simulink model "twoaxis_camera_gantry_start_work_project_Yejesh_final"  (R2025b)
settings: Solver=ode15s  StartTime=0.0  StopTime=60  MaxStep=1e-3  RelTol=1e-3  EnableMultiTasking=on
model workspace: external: MATLAB File gantryParams.m (data not in the file)
undefined symbols (not defined in the file): endSupport, endSupportZ, fractalcoef, leadScrew, leadScrewZ, rail, railZ, runner, runnerZ, X, Y, Z
libraries: sm_lib x81, nesl_utility x14, sm_linear_actuator_lib x14, fl_lib x6, slpidlib x2, mspsensorlib x1
(part 1 of 4)
Description:
  | Using the Lead Screw Joint Block - Linear Actuator
  | 
  | This example illustrates the use of the Lead Screw Joint block to model a linear actuator. The Lead
  | Screw Joint block converts rotational motion at the Revolute Joint block to translational motion at
  | the four Cylindrical Joint blocks. The translational motion is specified as a motion input to a
  | cylindrical joint and the necessary actuator torque is automatically computed at the revolute joint.
settings Model: PacingRate=4  Creator=The MathWorks, Inc.  LastModifiedBy=yejes
settings SolverCC: AlgebraicLoopSolver=TrustRegion
settings DataIOCC: LimitDataPoints=on  SaveFormat=Array  ReturnWorkspaceOutputs=off
settings OptimizationCC: LifeSpan=inf
settings DebuggingCC: SolverPrmCheckMsg=warning  UnconnectedInputMsg=warning  UnconnectedOutputMsg=warning  UnconnectedLineMsg=warning  AllowSymbolicDim=off  SFUnexpectedBacktrackingDiag=warning  SFNoUnconditionalDefaultTransitionDiag=warning  SFExecutionAtInitializationDiag=none  ArithmeticOperatorsInVariantConditions=warning
settings HardwareCC: ProdBitPerPointer=32.0  ProdBitPerSizeT=32.0  ProdBitPerPtrDiffT=32.0  ProdLargestAtomicFloat=None  ProdIntDivRoundTo=Undefined  ProdEndianess=Unspecified  ProdWordSize=32.0  ProdHWDeviceType=32-bit Generic
settings ModelReferenceCC: EnableRefExpFcnMdlSchedulingChecks=on  PropagateSignalLabelsOutOfModel=off
settings SFSimCC: SimUseLocalCustomCode=off  CustomCodeUndefinedFunction=UseInterfaceOnly
settings RTWCC: RTWUseLocalCustomCode=off  GPUComputeCapability=3.5  DLArmComputeVersion=19.05
settings CodeAppCC: StateflowObjectComments=on
settings GRTTargetCC: TargetLangStandard=C89/C90 (ANSI)
settings ConfigComp: CovMetricSettings=dw  CovSaveCumulativeToWorkspaceVar=on  CovSaveSingleToWorkspaceVar=on  CovExternalEMLEnable=off  CovSFcnEnable=off
settings SimscapeCC: SimscapeNormalizeSystem=off
settings ConfigurationSet: Description=SimMechanics 2G
settings DiagnosticsConfigSet: SimMechanicsUnconnectedFramePorts=none
settings ExplorerConfigSet: InternalSimMechanicsExplorerSettings="<ExplorerConfiguration><canonicalview>default</canonicalview><AnimationSetting><BasePlaybackSpeed>1.0</BasePlaybackSpeed><PlaybackSpeedFactor>1.0</PlaybackSpeedFactor></AnimationSetting><TilePanel><TileInfo><Tiles Columns=\"1\" Count=\"1\" Rows=\"1\"><Column Weight=\"1\"/><Row Weight=\"1\"/><Tile Height=\"1\" Width=\"1\" X=\"0\" Y=\"0\"/></Tiles></TileInfo><SceneInfo><SceneViewer><BGColor><R>1</R><G>1</G><B>1</B></BGColor><Camera><DoPerspective>off</DoPerspective><Position><X>0.577350260811389404</X><Y>-0.277350261388458308</Y><Z>0.937350262073923357</Z></Position><Center><X>-8.37823641020030152e-09</X><Y>0.300000007801167534</Y><Z>0.35999999288429757</Z></Center><Up><X>-0.408248290463863073</X><Y>0.408248290463863073</Y><Z>0.816496580927726145</Z></Up><ViewLimDist>1</ViewLimDist><YLim>0.483570086956024159</YLim><XLim>0.367001870038164535</XLim></Camera></SceneViewer></SceneInfo></TilePanel><MechEditorPanel><Cameras/><GfxPanelCameraMap/><VideoCreator><PlaybackSpeedRatio>1.0</PlaybackSpeedRatio><FrameRate>30</FrameRate><VideoFormat>Motion JPEG AVI</VideoFormat><FrameSize>auto</FrameSize></VideoCreator></MechEditorPanel></ExplorerConfiguration>"

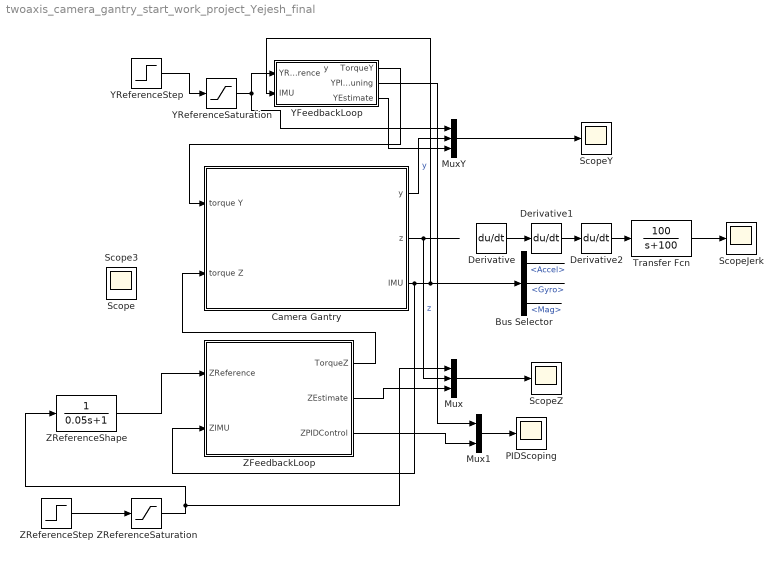
== system twoaxis_camera_gantry_start_work_project_Yejesh_final ==
  "\tCamera Gantry" : Subsystem
      mask Display: image('$imagefile'); % Use "Edit Image" on toolstrip to change.
  Bus Selector : BusSelector  OutputSignals=Accel,Gyro,Mag
  Derivative : Derivative
  Derivative1 : Derivative
  Derivative2 : Derivative
  Mux : Mux  Inputs=3
  Mux1 : Mux  Inputs=2
  MuxY : Mux  Inputs=3
  PIDScoping : Scope
      settings: ActiveDisplayYMinimum=-23.035365801646694  ActiveDisplayYMaximum=17.371677932919315  DataLoggingVariableName=ScopeData8
  ScopeJerk : Scope
  ScopeY : Scope
      settings: ActiveDisplayYMinimum=-0.074128762499999987  ActiveDisplayYMaximum=0.6671588625  DataLoggingVariableName=ScopeData2
  ScopeZ : Scope
      settings: ActiveDisplayYMinimum=-0.14165423833378787  ActiveDisplayYMaximum=0.64811641951018473  DataLoggingVariableName=ScopeData3
  Transfer Fcn : TransferFcn  Numerator=[100]  Denominator=[1 100]
  YFeedbackLoop : Subsystem
      settings: PortSchema="{\"entries\":[{\"content\":{\"sides\":[{\"content\":{\"connectorIds\":[\"In1\",\"In2\"]},\"type\":\"ConnectorPlacement.EquallySpacedRectSide\",\"uuid\":\"2f6c7822-fa00-4de6-9e32-64451994c035\"},{\"content\":{\"connectorIds\":[\"Out1\",\"Out2\",\"Out3\"],\"side\":\"RIGHT\"},\"type\":\"ConnectorPlacement.EquallySpacedRectSide\",\"uuid\":\"522d5529-44ef-4061-9e28-ddd46f5bc78d\"},{\"content\":{\"connectorIds\":[\"In3\"],\"side\":\"TOP\"},\"type\":\"ConnectorPlacement.EquallySpacedRectSide\",\"uuid\":\"f2a467b7-c03a-4305-9c34-f8fdeacd5866\"}]},\"type\":\"ConnectorPlacement.EquallySpacedConnector\",\"uuid\":\"6b65950b-cfc7-46ba-97f3-5f54aada1479\"}],\"packageUris\":[\"http://schema.mathworks.com/mf0/Connector/R2020b\"],\"version\":\"1.0\"}"
  YReferenceSaturation : Saturate  UpperLimit=0.75  LowerLimit=0
  YReferenceStep : Step  Time=0.5  Before=0.3  After=0.35  SampleTime=0
  ZFeedbackLoop : Subsystem
  ZReferenceSaturation : Saturate  UpperLimit=0.4  LowerLimit=0
  ZReferenceShape : TransferFcn  Denominator=[0.05 1]
  ZReferenceStep : Step  Time=0.5  Before=0.20  After=0.25  SampleTime=0
  Scope : Scope
      settings: ActiveDisplayYMinimum=-5.6117722223923652  ActiveDisplayYMaximum=5.5774668558867786  DataLoggingVariableName=ScopeData4
  Scope3 : Scope
      settings: ActiveDisplayYMinimum=0.1911  ActiveDisplayYMaximum=0.2439
  wires:
  "\tCamera Gantry"/3(IMU) -> ZFeedbackLoop/2(ZIMU), YFeedbackLoop/2(IMU), Bus Selector/1
  Bus Selector/1 -> ?  "<Accel>"
  Bus Selector/2 -> ?  "<Gyro>"
  Bus Selector/3 -> ?  "<Mag>"
  "\tCamera Gantry"/2(z) -> Mux/2  "z"
  YReferenceStep/1 -> YReferenceSaturation/1
  YReferenceSaturation/1 -> YFeedbackLoop/1(YReference), MuxY/1
  ZReferenceStep/1 -> ZReferenceSaturation/1
  ZReferenceSaturation/1 -> Mux/1, ZReferenceShape/1
  YFeedbackLoop/1(TorqueY) -> "\tCamera Gantry"/1(torque Y)
  ZReferenceShape/1 -> ZFeedbackLoop/1(ZReference)
  ZFeedbackLoop/1(TorqueZ) -> "\tCamera Gantry"/2(torque Z)
  Derivative/1 -> Derivative1/1
  Derivative1/1 -> Derivative2/1
  Derivative2/1 -> Transfer Fcn/1
  Transfer Fcn/1 -> ScopeJerk/1
  "\tCamera Gantry"/1(y) -> MuxY/2  "y"
  YFeedbackLoop/3(YEstimate) -> MuxY/3
  MuxY/1 -> ScopeY/1
  Mux/1 -> ScopeZ/1
  ZFeedbackLoop/2(ZEstimate) -> Mux/3
  Mux1/1 -> PIDScoping/1
  ZFeedbackLoop/3(ZPIDControl) -> Mux1/2
  YFeedbackLoop/2(YPIDTuning) -> Mux1/1

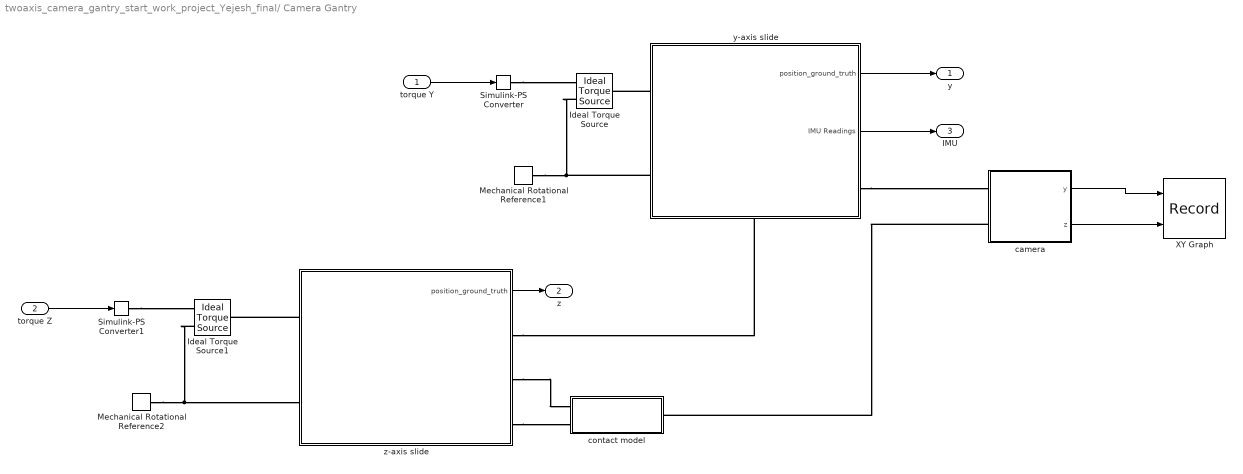
== system twoaxis_camera_gantry_start_work_project_Yejesh_final/	Camera Gantry ==
  torque Y : Inport
  torque Z : Inport  Port=2
  Ideal Torque Source : fl_lib/Mechanical/Mechanical Sources/Ideal Torque Source
  Ideal Torque Source1 : fl_lib/Mechanical/Mechanical Sources/Ideal Torque Source
  Mechanical Rotational Reference1 : fl_lib/Mechanical/Rotational Elements/Mechanical Rotational Reference
  Mechanical Rotational Reference2 : fl_lib/Mechanical/Rotational Elements/Mechanical Rotational Reference
  Simulink-PS Converter : nesl_utility/Simulink-PS Converter  PhysicalDomain=network_engine_domain  SubClassName=ps_input  LeftPortType=input  RightPortType=output  PseudoPeriodic=off  Frequencies=[]  NoiseDistribution=none  NoiseParameters=[]  Unit=1  AffineConversion=off  FilteringAndDerivatives=provide  SimscapeFilterOrder=1  InputFilterTimeConstant=0.001  UdotUserProvided=0
  Simulink-PS Converter1 : nesl_utility/Simulink-PS Converter  PhysicalDomain=network_engine_domain  SubClassName=ps_input  LeftPortType=input  RightPortType=output  PseudoPeriodic=off  Frequencies=[]  NoiseDistribution=none  NoiseParameters=[]  Unit=1  AffineConversion=off  FilteringAndDerivatives=provide  SimscapeFilterOrder=1  InputFilterTimeConstant=0.001  UdotUserProvided=0
  XY Graph : Record  NumPorts=2.0  FileSettingsInternal="{\"entries\":[{\"content\":{\"excelSettings\":{\"content\":{},\"type\":\"Streamout.ExcelSettings\"},\"parquetSettings\":{\"content\":{},\"type\":\"Streamout.ParquetSettings\"}},\"type\":\"Streamout.FileSettingStorage\",\"uuid\":\"\"}],\"packageUris\":[\"http:\\/\\/schema.mathworks.com\\/mf0\\/streamout_blocks\\/R2020a\"],\"version\":\"1.0\"}"  FrameSettings=[0, 0]  Layout=[1 1]  SignalsInternal="{\"entries\":[{\"content\":{\"signals\":[{\"content\":{\"blockPath\":[],\"dimensions\":[1],\"domain\":\"\",\"lineColor\":\"#a2142f\",\"plots\":[ 1 ],\"port\":1,\"sid\":[\"\"],\"signalID\":1,\"signalName\":\"camera:1\"},\"type\":\"RecordBlkView.Signal\",\"uuid\":\"\"},{\"content\":{\"blockPath\":[],\"dimensions\":[1],\"domain\":\"\",\"lineColor\":\"#139fff\",\"plots\":[ 1 ],\"port\":2,\"sid\":[\"\"],\"signalID\":2,\"signalName\":\"camera:2\"},\"type\":\"RecordBlkView.Signal\",\"uuid\":\"\"}]},\"type\":\"RecordBlkView.InputSignals\",\"uuid\":\"\"}],\"packageUris\":[\"http:\\/\\/schema.mathworks.com\\/mf0\\/streamout_blocks\\/R2020a\"],\"version\":\"1.0\"}"  VisualizationBindings="{\"xyplotplugin\":{\"info\":[{\"series\":[{\"bindingParametersList\":[{\"parameter\":\"X-Axis\",\"signalID\":1,\"signalName\":\"camera:1\"},{\"parameter\":\"Y-Axis\",\"signalID\":2,\"signalName\":\"camera:2\"}],\"seriesID\":0}],\"subplotID\":1}]}}"  CompatibilityTag=XY
  camera : Subsystem
      mask Display: image('$imagefile'); % Use "Edit Image" on toolstrip to change.
  contact model : Subsystem
  y-axis slide : Subsystem
      settings: PortSchema="{\"entries\":[{\"content\":{\"sides\":[{\"content\":{\"connectorIds\":[\"LConn1\",\"LConn2\"]},\"type\":\"ConnectorPlacement.EquallySpacedRectSide\",\"uuid\":\"3f377b63-bc87-4e06-8b63-1d64c166b4f3\"},{\"content\":{\"connectorIds\":[\"Out1\",\"Out2\",\"RConn1\"],\"side\":\"RIGHT\"},\"type\":\"ConnectorPlacement.EquallySpacedRectSide\",\"uuid\":\"3affb14a-8bdc-4f8f-893e-0f417901967e\"},{\"content\":{\"connectorIds\":[],\"side\":\"TOP\"},\"type\":\"ConnectorPlacement.EquallySpacedRectSide\",\"uuid\":\"c82e62d7-ab85-41ce-b1ad-21607245c47e\"},{\"content\":{\"connectorIds\":[\"RConn2\"],\"side\":\"BOTTOM\"},\"type\":\"ConnectorPlacement.EquallySpacedRectSide\",\"uuid\":\"9d54362b-4991-4bea-87e6-d83ba5b68b2b\"}]},\"type\":\"ConnectorPlacement.EquallySpacedConnector\",\"uuid\":\"4017ed31-76af-4f0f-8b41-874461299965\"}],\"packageUris\":[\"http://schema.mathworks.com/mf0/Connector/R2020b\"],\"version\":\"1.0\"}"
      mask Display: image('$imagefile'); % Use "Edit Image" on toolstrip to change.
  z-axis slide : Subsystem
      mask Display: image('$imagefile'); % Use "Edit Image" on toolstrip to change.
  y : Outport
  z : Outport  Port=2
  IMU : Outport  Port=3
  wires:
  camera/1(y) -> XY Graph/1
  y-axis slide/1(position_ground_truth) -> y/1
  y-axis slide/2(IMU Readings) -> IMU/1
  z-axis slide/1(position_ground_truth) -> z/1
  camera/2(z) -> XY Graph/2
  torque Y/1 -> Simulink-PS Converter/1
  torque Z/1 -> Simulink-PS Converter1/1
  connections:
  y-axis slide/LConn1 -- Ideal Torque Source/LConn1
  y-axis slide/RConn1 -- camera/LConn1
  z-axis slide/LConn1 -- Ideal Torque Source1/LConn1
  Ideal Torque Source1/RConn2 -- Mechanical Rotational Reference2/LConn1 -- z-axis slide/LConn2
  z-axis slide/RConn1 -- y-axis slide/RConn2
  z-axis slide/RConn2 -- contact model/LConn1
  z-axis slide/RConn3 -- contact model/LConn2
  camera/LConn2 -- contact model/RConn1
  Mechanical Rotational Reference1/LConn1 -- Ideal Torque Source/RConn2 -- y-axis slide/LConn2
  Simulink-PS Converter/RConn1 -- Ideal Torque Source/RConn1
  Simulink-PS Converter1/RConn1 -- Ideal Torque Source1/RConn1

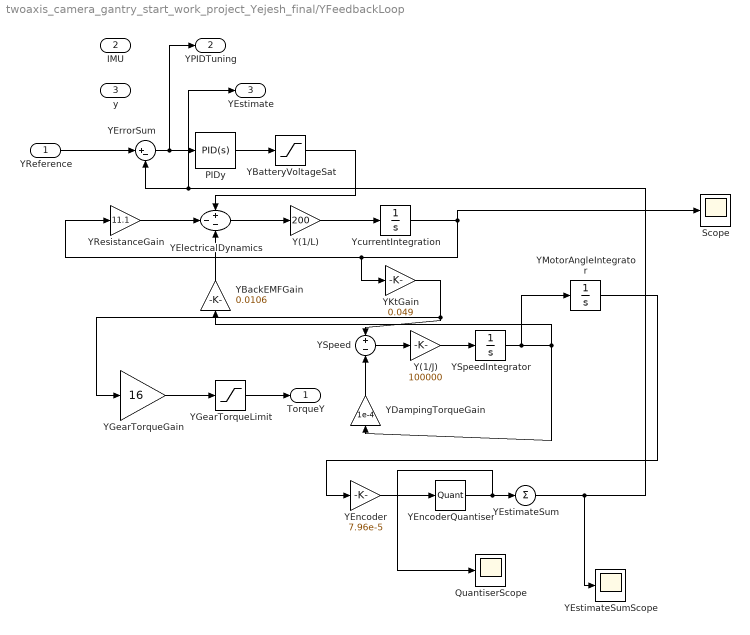
== system twoaxis_camera_gantry_start_work_project_Yejesh_final/YFeedbackLoop ==
  YReference : Inport
  IMU : Inport  Port=2
  y : Inport  Port=3
  PIDy : slpidlib/PID Controller  Controller=PID  Form=Parallel  TimeDomain=Continuous-time  UseExternalTs=off  SampleTime=-1  IntegratorMethod=Forward Euler  FilterMethod=Forward Euler  ControllerParametersSource=internal  P=30  I=10  UseKiTs=off  D=2  UseExternalDerivativeSource=off  N=100  UseFilter=on  TunerSelectOption=Transfer Function Based (PID Tuner App)  InitialConditionSource=internal  InitialConditionForIntegrator=0  InitialConditionForFilter=0  DifferentiatorICPrevScaledInput=0  ExternalReset=none  TrackingMode=off  Kt=1  LimitOutput=off  SatLimitsSource=internal  UpperSaturationLimit=inf  LowerSaturationLimit=-inf  LinearizeAsGain=on  AntiWindupMode=none  Kb=1  LimitIntegrator=off  UpperIntegratorSaturationLimit=inf  LowerIntegratorSaturationLimit=-inf  POutMin=[]  POutMax=[]  IOutMin=[]  IOutMax=[]  DOutMin=[]  DOutMax=[]  NOutMin=[]  NOutMax=[]  SumOutMin=[]  SumOutMax=[]  SaturationOutMin=[]  SaturationOutMax=[]  PParamMin=[]  PParamMax=[]  IParamMin=[]  IParamMax=[]  DParamMin=[]  DParamMax=[]  NParamMin=[]  NParamMax=[]  KbParamMin=[]  KbParamMax=[]  KtParamMin=[]  KtParamMax=[]  KbOutMin=[]  KbOutMax=[]  KtOutMin=[]  KtOutMax=[]  IntegratorOutMin=[]  IntegratorOutMax=[]  FilterOutMin=[]  FilterOutMax=[]  SumI1OutMin=[]  SumI1OutMax=[]  SumI2OutMin=[]  SumI2OutMax=[]  SumI3OutMin=[]  SumI3OutMax=[]  SumI4OutMin=[]  SumI4OutMax=[]  SumDOutMin=[]  SumDOutMax=[]  DifferentiatorOutMin=[]  DifferentiatorOutMax=[]  FilterDiffOutCoefMin=[]  FilterDiffOutCoefMax=[]  ReciprocalOutMin=[]  ReciprocalOutMax=[]  SumDenOutMin=[]  SumDenOutMax=[]  SumNumOutMin=[]  SumNumOutMax=[]  DivideOutMin=[]  DivideOutMax=[]  UdiffTsProdOutMin=[]  UdiffTsProdOutMax=[]  NTsProdOutMin=[]  NTsProdOutMax=[]  UintegralTsProdOutMin=[]  UintegralTsProdOutMax=[]  UngainTsProdOutMin=[]  UngainTsProdOutMax=[]  ClampingZeroOutDataTypeStr=Inherit: Inherit via back propagation  ClampingZeroOutMin=[]  ClampingZeroOutMax=[]  FilterDenConstantOutDataTypeStr=Inherit: Inherit via back propagation  FilterDenConstantOutMin=[]  FilterDenConstantOutMax=[]  PCopyOutDataTypeStr=Inherit: Inherit via back propagation  PCopyOutMin=[]  PCopyOutMax=[]  NCopyOutDataTypeStr=Inherit: Inherit via back propagation  NCopyOutMin=[]  NCopyOutMax=[]  IntegratorContinuousStateAttributes=''  IntegratorStateMustResolveToSignalObject=off  IntegratorRTWStateStorageClass=Auto  FilterContinuousStateAttributes=''  FilterStateMustResolveToSignalObject=off  FilterRTWStateStorageClass=Auto  ParallelPVariant=InternalParameters  IdealPVariant=Disabled  IVariant=InternalParameters  DVariant=InternalParameters  IntegratorVariant=Continuous  SatVariant=Disabled  AWVariant=Passthrough  PCopyVariant=Disabled  TRVariant=Disabled  FdbkBlocksVariant=Forward  IdealPFdbkVariant=Disabled  SatFdbkVariant=Disabled  DerivativeFilterVariant=ContFilter  NVariant=InternalParameters  NCopyVariant=Disabled  FilterICVariant=InternalICsFilter  IntegratorICVariant=InternalICs  ExternalResetVariant=Disabled  TRSumVariant=Passthrough  SumFdbkVariant=Disabled  SumVariant=Sum_PID  TsampFilterVariant=InternalTs  TsampNgainVariant=Passthrough  TsampIntegralVariant=Disabled_SignalSpec  ExternalSaturationOutDataTypeStr=Inherit: Same as second input  DerivativeSourceVariant=ErrorSignal  PreIntVariant=InternalPreInt
  QuantiserScope : Scope
      settings: DataLoggingVariableName=ScopeData5
  Scope : Scope
      settings: ActiveDisplayYMinimum=-0.89118502896327889  ActiveDisplayYMaximum=1.198287194267555  DataLoggingVariableName=ScopeData7
  Y(1/J) : Gain  Gain=100000
  Y(1/L) : Gain  Gain=200
  YBackEMFGain : Gain  Gain=0.0106
  YBatteryVoltageSat : Saturate  UpperLimit=11.1  LowerLimit=-11.1
  YDampingTorqueGain : Gain  Gain=1e-4
  YElectricalDynamics : Sum  Inputs=+--
  YEncoder : Gain  Gain=7.96e-5
  YEncoderQuantiser : Quantizer  QuantizationInterval=2.083e-5
  YErrorSum : Sum  Inputs=|+-
  YEstimateSum : Sum  Inputs=+
  YEstimateSumScope : Scope
      settings: ActiveDisplayYMinimum=-8.828451733084659  ActiveDisplayYMaximum=8.4483002375448635  DataLoggingVariableName=ScopeData6
  YGearTorqueGain : Gain  Gain=16
  YGearTorqueLimit : Saturate  UpperLimit=0.784  LowerLimit=-0.784
  YKtGain : Gain  Gain=0.049
  YMotorAngleIntegrator : Integrator
  YResistanceGain : Gain  Gain=11.1
  YSpeed : Sum  Inputs=+-
  YSpeedIntegrator : Integrator
  YcurrentIntegration : Integrator
  TorqueY : Outport
  YPIDTuning : Outport  Port=2
  YEstimate : Outport  Port=3
  wires:
  YElectricalDynamics/1 -> Y(1/L)/1
  YcurrentIntegration/1 -> YResistanceGain/1, YKtGain/1, Scope/1
  YBackEMFGain/1 -> YElectricalDynamics/3
  YResistanceGain/1 -> YElectricalDynamics/2
  YSpeedIntegrator/1 -> YDampingTorqueGain/1, YBackEMFGain/1, YMotorAngleIntegrator/1
  YKtGain/1 -> YGearTorqueGain/1, YSpeed/1
  YErrorSum/1 -> YPIDTuning/1, PIDy/1
  YBatteryVoltageSat/1 -> YElectricalDynamics/1
  PIDy/1 -> YBatteryVoltageSat/1
  Y(1/J)/1 -> YSpeedIntegrator/1
  Y(1/L)/1 -> YcurrentIntegration/1
  YDampingTorqueGain/1 -> YSpeed/2
  YSpeed/1 -> Y(1/J)/1
  YReference/1 -> YErrorSum/1
  YGearTorqueGain/1 -> YGearTorqueLimit/1
  YGearTorqueLimit/1 -> TorqueY/1
  YMotorAngleIntegrator/1 -> YEncoder/1
  YEncoder/1 -> YEncoderQuantiser/1
  YEncoderQuantiser/1 -> QuantiserScope/1, YEstimateSum/1
  YEstimateSum/1 -> YEstimateSumScope/1, YEstimate/1, YErrorSum/2

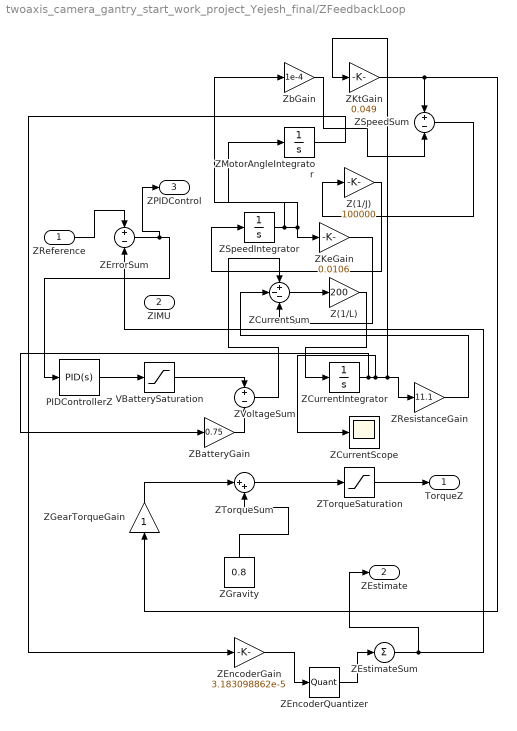
== system twoaxis_camera_gantry_start_work_project_Yejesh_final/ZFeedbackLoop ==
  ZReference : Inport
  ZIMU : Inport  Port=2
  PIDControllerZ : slpidlib/PID Controller  Controller=PID  Form=Parallel  TimeDomain=Continuous-time  UseExternalTs=off  SampleTime=-1  IntegratorMethod=Forward Euler  FilterMethod=Forward Euler  ControllerParametersSource=internal  P=50  I=30  UseKiTs=off  D=2  UseExternalDerivativeSource=off  N=100  UseFilter=on  TunerSelectOption=Transfer Function Based (PID Tuner App)  InitialConditionSource=internal  InitialConditionForIntegrator=0  InitialConditionForFilter=0  DifferentiatorICPrevScaledInput=0  ExternalReset=none  TrackingMode=off  Kt=1  LimitOutput=off  SatLimitsSource=internal  UpperSaturationLimit=inf  LowerSaturationLimit=-inf  LinearizeAsGain=on  AntiWindupMode=none  Kb=1  LimitIntegrator=off  UpperIntegratorSaturationLimit=inf  LowerIntegratorSaturationLimit=-inf  POutMin=[]  POutMax=[]  IOutMin=[]  IOutMax=[]  DOutMin=[]  DOutMax=[]  NOutMin=[]  NOutMax=[]  SumOutMin=[]  SumOutMax=[]  SaturationOutMin=[]  SaturationOutMax=[]  PParamMin=[]  PParamMax=[]  IParamMin=[]  IParamMax=[]  DParamMin=[]  DParamMax=[]  NParamMin=[]  NParamMax=[]  KbParamMin=[]  KbParamMax=[]  KtParamMin=[]  KtParamMax=[]  KbOutMin=[]  KbOutMax=[]  KtOutMin=[]  KtOutMax=[]  IntegratorOutMin=[]  IntegratorOutMax=[]  FilterOutMin=[]  FilterOutMax=[]  SumI1OutMin=[]  SumI1OutMax=[]  SumI2OutMin=[]  SumI2OutMax=[]  SumI3OutMin=[]  SumI3OutMax=[]  SumI4OutMin=[]  SumI4OutMax=[]  SumDOutMin=[]  SumDOutMax=[]  DifferentiatorOutMin=[]  DifferentiatorOutMax=[]  FilterDiffOutCoefMin=[]  FilterDiffOutCoefMax=[]  ReciprocalOutMin=[]  ReciprocalOutMax=[]  SumDenOutMin=[]  SumDenOutMax=[]  SumNumOutMin=[]  SumNumOutMax=[]  DivideOutMin=[]  DivideOutMax=[]  UdiffTsProdOutMin=[]  UdiffTsProdOutMax=[]  NTsProdOutMin=[]  NTsProdOutMax=[]  UintegralTsProdOutMin=[]  UintegralTsProdOutMax=[]  UngainTsProdOutMin=[]  UngainTsProdOutMax=[]  ClampingZeroOutDataTypeStr=Inherit: Inherit via back propagation  ClampingZeroOutMin=[]  ClampingZeroOutMax=[]  FilterDenConstantOutDataTypeStr=Inherit: Inherit via back propagation  FilterDenConstantOutMin=[]  FilterDenConstantOutMax=[]  PCopyOutDataTypeStr=Inherit: Inherit via back propagation  PCopyOutMin=[]  PCopyOutMax=[]  NCopyOutDataTypeStr=Inherit: Inherit via back propagation  NCopyOutMin=[]  NCopyOutMax=[]  IntegratorContinuousStateAttributes=''  IntegratorStateMustResolveToSignalObject=off  IntegratorRTWStateStorageClass=Auto  FilterContinuousStateAttributes=''  FilterStateMustResolveToSignalObject=off  FilterRTWStateStorageClass=Auto  ParallelPVariant=InternalParameters  IdealPVariant=Disabled  IVariant=InternalParameters  DVariant=InternalParameters  IntegratorVariant=Continuous  SatVariant=Disabled  AWVariant=Passthrough  PCopyVariant=Disabled  TRVariant=Disabled  FdbkBlocksVariant=Forward  IdealPFdbkVariant=Disabled  SatFdbkVariant=Disabled  DerivativeFilterVariant=ContFilter  NVariant=InternalParameters  NCopyVariant=Disabled  FilterICVariant=InternalICsFilter  IntegratorICVariant=InternalICs  ExternalResetVariant=Disabled  TRSumVariant=Passthrough  SumFdbkVariant=Disabled  SumVariant=Sum_PID  TsampFilterVariant=InternalTs  TsampNgainVariant=Passthrough  TsampIntegralVariant=Disabled_SignalSpec  ExternalSaturationOutDataTypeStr=Inherit: Same as second input  DerivativeSourceVariant=ErrorSignal  PreIntVariant=InternalPreInt
  VBatterySaturation : Saturate  UpperLimit=11.1  LowerLimit=-11.1
  Z(1/J) : Gain  Gain=100000
  Z(1/L) : Gain  Gain=200
  ZBatteryGain : Gain  Gain=0.75
  ZCurrentIntegrator : Integrator
  ZCurrentScope : Scope
      settings: ActiveDisplayYMinimum=-26.108293801727836  ActiveDisplayYMaximum=18.44047191563121  DataLoggingVariableName=ScopeData9
  ZCurrentSum : Sum  Inputs=+--
  ZEncoderGain : Gain  Gain=3.183098862e-5
  ZEncoderQuantizer : Quantizer  QuantizationInterval=8.33e-6
  ZErrorSum : Sum  Inputs=+-
  ZEstimateSum : Sum  Inputs=+
  ZGearTorqueGain : Gain
  ZGravity : Constant  Value=0.8
  ZKeGain : Gain  Gain=0.0106
  ZKtGain : Gain  Gain=0.049
  ZMotorAngleIntegrator : Integrator
  ZResistanceGain : Gain  Gain=11.1
  ZSpeedIntegrator : Integrator
  ZSpeedSum : Sum  Inputs=+-
  ZTorqueSaturation : Saturate  UpperLimit=1.96  LowerLimit=-1.96
  ZTorqueSum : Sum  Inputs=|++
  ZVoltageSum : Sum  Inputs=+-
  ZbGain : Gain  Gain=1e-4
  TorqueZ : Outport
  ZEstimate : Outport  Port=2
  ZPIDControl : Outport  Port=3
  wires:
  ZReference/1 -> ZErrorSum/1
  ZErrorSum/1 -> ZPIDControl/1, PIDControllerZ/1
  PIDControllerZ/1 -> VBatterySaturation/1
  VBatterySaturation/1 -> ZVoltageSum/1
  ZBatteryGain/1 -> ZVoltageSum/2
  ZVoltageSum/1 -> ZCurrentSum/1
  ZCurrentIntegrator/1 -> ZBatteryGain/1, ZCurrentScope/1, ZKtGain/1, ZResistanceGain/1
  ZResistanceGain/1 -> ZCurrentSum/2
  ZKeGain/1 -> ZCurrentSum/3
  ZCurrentSum/1 -> Z(1/L)/1
  Z(1/L)/1 -> ZCurrentIntegrator/1
  ZSpeedIntegrator/1 -> ZbGain/1, ZKeGain/1, ZMotorAngleIntegrator/1
  ZKtGain/1 -> ZGearTorqueGain/1, ZSpeedSum/1
  ZbGain/1 -> ZSpeedSum/2
  ZSpeedSum/1 -> Z(1/J)/1
  Z(1/J)/1 -> ZSpeedIntegrator/1
  ZGearTorqueGain/1 -> ZTorqueSum/1
  ZGravity/1 -> ZTorqueSum/2
  ZTorqueSum/1 -> ZTorqueSaturation/1
  ZMotorAngleIntegrator/1 -> ZEncoderGain/1
  ZEncoderGain/1 -> ZEncoderQuantizer/1
  ZEncoderQuantizer/1 -> ZEstimateSum/1
  ZEstimateSum/1 -> ZEstimate/1, ZErrorSum/2
  ZTorqueSaturation/1 -> TorqueZ/1

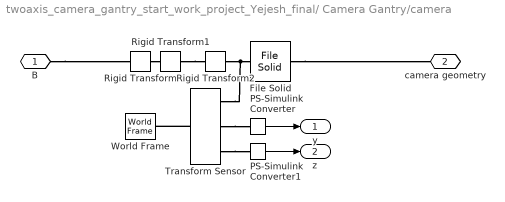
== system twoaxis_camera_gantry_start_work_project_Yejesh_final/	Camera Gantry/camera ==
  File Solid : sm_lib/Body Elements/File Solid  ExtGeomFileName=canon.stl  UnitType=Custom  ExtGeomFileUnits=mm  StepReaderType=HEX  ExportConvexHullGeometry=on  InertiaType=CalculateFromGeometry  BasedOnType=Density  Density=5  DensityUnits=g/cm^3  Mass=15  MassUnits=kg  CenterOfMass=[0 0 0]  CenterOfMassUnits=m  MomentsOfInertia=[1 1 1]  MomentsOfInertiaUnits=kg*m^2  ProductsOfInertia=[0 0 0]  ProductsOfInertiaUnits=kg*m^2  GraphicType=FromGeometry  MarkerShape=Sphere  MarkerSize=10  GraphicVisPropType=SimpleVisualProperties  GraphicDiffuseColor=[0.5 0.5 0.5]  GraphicOpacity=1.0  GraphicSpecularColor=[0.5 0.5 0.5 1.0]  GraphicAmbientColor=[0.15 0.15 0.15 1.0]  GraphicEmissiveColor=[0.0 0.0 0.0 1.0]  GraphicShininess=75  DoExposeReferenceFrame=off  SerializedFrames=<Frames><Frame><Id>Frame1</Id><Value><Name>F1</Name><Origin><Source>CenterOfMassFrame</Source><FeatureName></FeatureName></Origin><PrimaryAxis><DefinedDirection>+Z</DefinedDirection><Source>ReferenceFrame</Source><SourceDirection>+Z</SourceDirection><FeatureName></FeatureName></PrimaryAxis><SecondaryAxis><DefinedDirection>+X</DefinedDirection><Source>ReferenceFrame</Source><SourceDirection>+X</SourceDirection><FeatureName></FeatureName></SecondaryAxis></Value></Frame></Frames>
  PS-Simulink Converter : nesl_utility/PS-Simulink Converter  PhysicalDomain=network_engine_domain  SubClassName=ps_output  LeftPortType=input  RightPortType=output  PseudoPeriodic=off  Frequencies=[]  VectorFormat=1-D array  Unit=inherit  AffineConversion=off
  PS-Simulink Converter1 : nesl_utility/PS-Simulink Converter  PhysicalDomain=network_engine_domain  SubClassName=ps_output  LeftPortType=input  RightPortType=output  PseudoPeriodic=off  Frequencies=[]  VectorFormat=1-D array  Unit=inherit  AffineConversion=off
  Rigid Transform : sm_lib/Frames and Transforms/Rigid Transform  RotationMethod=StandardAxis  FollAlignAxisA=+X  BaseAlignAxisA=+Y  FollAlignAxisB=+Y  BaseAlignAxisB=+Z  RotationStandardAxis=-X  RotationAngle=90  RotationAngleUnits=deg  RotationArbitraryAxis=[0 0 1]  RotationSequenceAxes=FollowerAxes  RotationSequence=XYX  RotationSequenceAngles=[0 0 0]  RotationSequenceAnglesUnits=deg  RotationMatrix=[1 0 0; 0 1 0; 0 0 1]  Quaternion=[1 0 0 0]  TranslationMethod=None  TranslationCartesianOffset=[0 0 0]  TranslationCartesianOffsetUnits=m  TranslationStandardAxis=+Z  TranslationStandardOffset=0  TranslationStandardOffsetUnits=m  TranslationROffset=0  TranslationROffsetUnits=m  TranslationThetaOffset=0  TranslationThetaOffsetUnits=deg  TranslationZOffset=0  TranslationZOffsetUnits=m
  Rigid Transform1 : sm_lib/Frames and Transforms/Rigid Transform  RotationMethod=StandardAxis  FollAlignAxisA=+X  BaseAlignAxisA=+Y  FollAlignAxisB=+Y  BaseAlignAxisB=+Z  RotationStandardAxis=+Z  RotationAngle=90  RotationAngleUnits=deg  RotationArbitraryAxis=[0 0 1]  RotationSequenceAxes=FollowerAxes  RotationSequence=XYX  RotationSequenceAngles=[0 0 0]  RotationSequenceAnglesUnits=deg  RotationMatrix=[1 0 0; 0 1 0; 0 0 1]  Quaternion=[1 0 0 0]  TranslationMethod=None  TranslationCartesianOffset=[0 0 0]  TranslationCartesianOffsetUnits=m  TranslationStandardAxis=+Z  TranslationStandardOffset=0  TranslationStandardOffsetUnits=m  TranslationROffset=0  TranslationROffsetUnits=m  TranslationThetaOffset=0  TranslationThetaOffsetUnits=deg  TranslationZOffset=0  TranslationZOffsetUnits=m
  Rigid Transform2 : sm_lib/Frames and Transforms/Rigid Transform  RotationMethod=None  FollAlignAxisA=+X  BaseAlignAxisA=+Y  FollAlignAxisB=+Y  BaseAlignAxisB=+Z  RotationStandardAxis=+Z  RotationAngle=90  RotationAngleUnits=deg  RotationArbitraryAxis=[0 0 1]  RotationSequenceAxes=FollowerAxes  RotationSequence=XYX  RotationSequenceAngles=[0 0 0]  RotationSequenceAnglesUnits=deg  RotationMatrix=[1 0 0; 0 1 0; 0 0 1]  Quaternion=[1 0 0 0]  TranslationMethod=Cartesian  TranslationCartesianOffset=[0 -30 47]  TranslationCartesianOffsetUnits=mm  TranslationStandardAxis=+Z  TranslationStandardOffset=47  TranslationStandardOffsetUnits=mm  TranslationROffset=0  TranslationROffsetUnits=m  TranslationThetaOffset=0  TranslationThetaOffsetUnits=deg  TranslationZOffset=0  TranslationZOffsetUnits=m
  Transform Sensor : sm_lib/Frames and Transforms/Transform Sensor  MeasurementFrame=World  RotationSequence=XYX  SenseAngle=off  SenseAxis=off  SenseQ=off  SenseR=off  SenseRotationSequence=off  SenseOmegaX=off  SenseOmegaY=off  SenseOmegaZ=off  SenseOmega=off  SenseQDot=off  SenseRDot=off  SenseRotationSequenceDot=off  SenseAlphaX=off  SenseAlphaY=off  SenseAlphaZ=off  SenseAlpha=off  SenseQDDot=off  SenseRDDot=off  SenseX=off  SenseY=on  SenseZ=on  SenseXYZ=off  SenseRad=off  SenseAzim=off  SenseDist=off  SenseInc=off  SenseXDot=off  SenseYDot=off  SenseZDot=off  SenseXYZDot=off  SenseRadDot=off  SenseAzimDot=off  SenseDistDot=off  SenseIncDot=off  SenseXDDot=off  SenseYDDot=off  SenseZDDot=off  SenseXYZDDot=off  SenseRadDDot=off  SenseAzimDDot=off  SenseDistDDot=off  SenseIncDDot=off
  World Frame : sm_lib/Frames and Transforms/World Frame
  B : PMIOPort  Side=Left
  camera geometry : PMIOPort  Port=2  Side=Left
  y : Outport
  z : Outport  Port=2
  wires:
  PS-Simulink Converter/1 -> y/1
  PS-Simulink Converter1/1 -> z/1
  connections:
  Rigid Transform1/RConn1 -- Rigid Transform2/LConn1
  Rigid Transform2/RConn1 -- Transform Sensor/RConn1 -- File Solid/LConn1
  Rigid Transform/RConn1 -- Rigid Transform1/LConn1
  Transform Sensor/LConn1 -- World Frame/RConn1
  Transform Sensor/RConn2 -- PS-Simulink Converter/LConn1
  B/RConn1 -- Rigid Transform/LConn1
  Transform Sensor/RConn3 -- PS-Simulink Converter1/LConn1
  File Solid/RConn1 -- camera geometry/RConn1

== system twoaxis_camera_gantry_start_work_project_Yejesh_final/	Camera Gantry/contact model ==
  Spatial Contact Force : sm_lib/Forces and Torques/Spatial Contact Force  SenseSeparationDistance=off  NormalForceType=SmoothSpringDamper  NormalStiffness=1e7  NormalStiffnessUnits=N/m  NormalDamping=1e5  NormalDampingUnits=N/(m/s)  NormalTransitionRegionWidth=1e-4  NormalTransitionRegionWidthUnits=m  FrictionType=SmoothStickSlip  CoefficientOfStaticFriction=0.5  CoefficientOfDynamicFriction=0.3  FrictionalCriticalVelocity=1e-3  FrictionalCriticalVelocityUnits=m/s  SenseContactSignal=off  SensePenetrationDepth=off  SenseNormalVelocity=off  SenseTangentialVelocity=off  SensingForceTorqueDirection=BaseOnFollower  SensingForceTorqueResolutionFrame=ContactFrame  SenseNormalForce=off  SenseNormalForceMagnitude=off  SenseNormalTorque=off  SenseFrictionalForce=off  SenseFrictionalForceMagnitude=off  SenseFrictionalTorque=off  SenseTotalForce=off  SenseTotalTorque=off  SenseContactBaseRotation=off  SenseContactBaseTranslation=off  SenseContactFollowerRotation=off  SenseContactFollowerTranslation=off  ZeroCrossDetectContactStartAndEnd=off
  Spatial Contact Force1 : sm_lib/Forces and Torques/Spatial Contact Force  SenseSeparationDistance=off  NormalForceType=SmoothSpringDamper  NormalStiffness=1e6  NormalStiffnessUnits=N/m  NormalDamping=1e3  NormalDampingUnits=N/(m/s)  NormalTransitionRegionWidth=1e-4  NormalTransitionRegionWidthUnits=m  FrictionType=SmoothStickSlip  CoefficientOfStaticFriction=0.5  CoefficientOfDynamicFriction=0.3  FrictionalCriticalVelocity=1e-3  FrictionalCriticalVelocityUnits=m/s  SenseContactSignal=off  SensePenetrationDepth=off  SenseNormalVelocity=off  SenseTangentialVelocity=off  SensingForceTorqueDirection=BaseOnFollower  SensingForceTorqueResolutionFrame=ContactFrame  SenseNormalForce=off  SenseNormalForceMagnitude=off  SenseNormalTorque=off  SenseFrictionalForce=off  SenseFrictionalForceMagnitude=off  SenseFrictionalTorque=off  SenseTotalForce=off  SenseTotalTorque=off  SenseContactBaseRotation=off  SenseContactBaseTranslation=off  SenseContactFollowerRotation=off  SenseContactFollowerTranslation=off  ZeroCrossDetectContactStartAndEnd=off
  ceiling : PMIOPort  Side=Left
  wall : PMIOPort  Port=2  Side=Left
  camera : PMIOPort  Port=3  Side=Right
  connections:
  Spatial Contact Force1/LConn1 -- ceiling/RConn1
  Spatial Contact Force1/RConn1 -- Spatial Contact Force/RConn1 -- camera/RConn1
  Spatial Contact Force/LConn1 -- wall/RConn1
